simulink model "lab6"  (R2015a)
settings: Solver=ode45  StartTime=0.0  StopTime=500.0  MaxStep=0.2  RelTol=1e-3
values from neighbouring files (symbols this model uses):
  ddMax = 3    [lab6.m]
  deltaMax = 30    [lab6.m]
  fConst = 0    [lab6.m]
  K = 0.08    [lab6.m]
  Kaw = 2.604    [lab6.m]
  Kc = 1.04    [lab6.m]
  phiZad = 30    [lab6.m]
  Ti = 200    [lab6.m]
  Tr = 1    [lab6.m]
  Ts = 16.4    [lab6.m]
settings Model: Creator=vbox  LastModifiedBy=vbox
settings DataIOCC: InspectSignalLogs=on

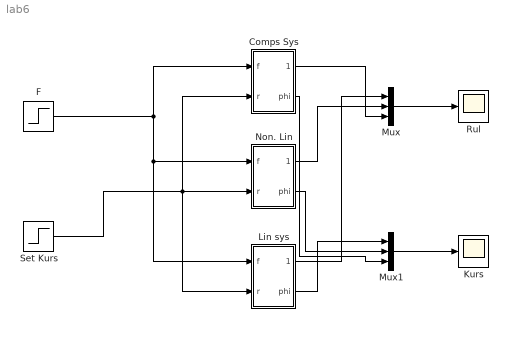
== system lab6 ==
  Comps Sys : Subsystem
  F : Step  After=fConst  SampleTime=0
  Kurs : Scope
      settings: SaveName=phi
  Lin sys : Subsystem
  Mux : Mux  Inputs=3
  Mux1 : Mux  Inputs=3
  Non. Lin : Subsystem
  Rul : Scope
      settings: TimeRange=100  YMin=0  YMax=400  SaveName=delta
  Set Kurs : Step  Time=0  After=phiZad  SampleTime=0
  wires:
  F/1 -> Non. Lin/1(f), Lin sys/1(f), Comps Sys/1(f)
  Set Kurs/1 -> Lin sys/2(r), Comps Sys/2(r), Non. Lin/2(r)
  Mux1/1 -> Kurs/1
  Mux/1 -> Rul/1
  Lin sys/1(delta) -> Mux/1
  Lin sys/2(phi) -> Mux1/1
  Non. Lin/1(delta) -> Mux/2
  Non. Lin/2(phi) -> Mux1/2
  Comps Sys/2(phi) -> Mux1/3
  Comps Sys/1(delta) -> Mux/3

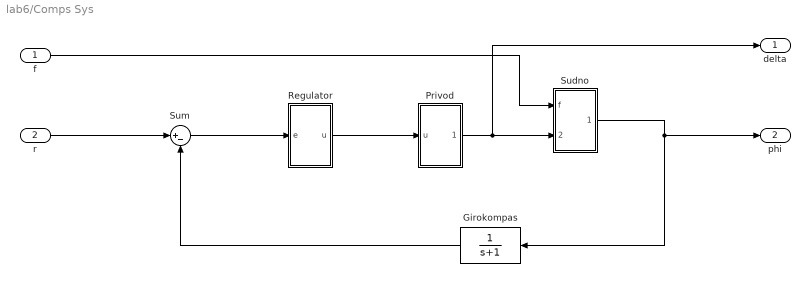
== system lab6/Comps Sys ==
  f : Inport
  r : Inport  Port=2
  Girokompas : TransferFcn  Denominator=[1 1]
  Privod : Subsystem
  Regulator : Subsystem
  Sudno : Subsystem
  Sum : Sum  Inputs=|+-
  delta : Outport
  phi : Outport  Port=2
  wires:
  Girokompas/1 -> Sum/2
  r/1 -> Sum/1
  Sudno/1(phi) -> phi/1, Girokompas/1
  Sum/1 -> Regulator/1(e)
  f/1 -> Sudno/1(f)
  Privod/1(delta) -> delta/1, Sudno/2(delta)
  Regulator/1(u) -> Privod/1(u)

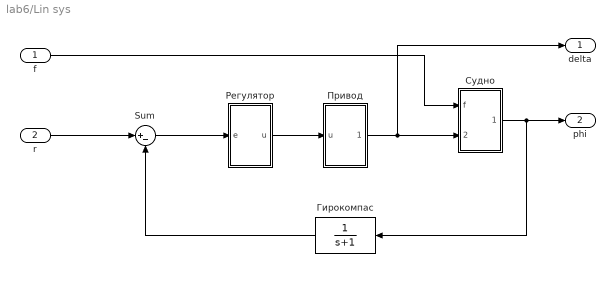
== system lab6/Lin sys ==
  f : Inport
  r : Inport  Port=2
  Sum : Sum  Inputs=|+-
  Гирокомпас : TransferFcn  Denominator=[1 1]
  Привод : Subsystem
  Регулятор : Subsystem
  Судно : Subsystem
  delta : Outport
  phi : Outport  Port=2
  wires:
  Гирокомпас/1 -> Sum/2
  r/1 -> Sum/1
  Судно/1(phi) -> phi/1, Гирокомпас/1
  Sum/1 -> Регулятор/1(e)
  f/1 -> Судно/1(f)
  Привод/1(delta) -> delta/1, Судно/2(delta)
  Регулятор/1(u) -> Привод/1(u)

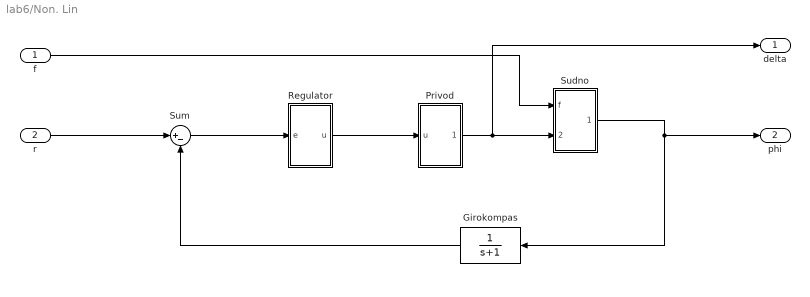
== system lab6/Non. Lin ==
  f : Inport
  r : Inport  Port=2
  Girokompas : TransferFcn  Denominator=[1 1]
  Privod : Subsystem
  Regulator : Subsystem
  Sudno : Subsystem
  Sum : Sum  Inputs=|+-
  delta : Outport
  phi : Outport  Port=2
  wires:
  Girokompas/1 -> Sum/2
  r/1 -> Sum/1
  Sudno/1(phi) -> phi/1, Girokompas/1
  Sum/1 -> Regulator/1(e)
  f/1 -> Sudno/1(f)
  Privod/1(delta) -> delta/1, Sudno/2(delta)
  Regulator/1(u) -> Privod/1(u)

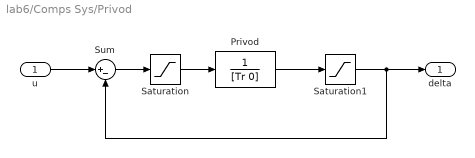
== system lab6/Comps Sys/Privod ==
  u : Inport
  Privod : TransferFcn  Denominator=[Tr 0]
  Saturation : Saturate  UpperLimit=Tr*ddMax  LowerLimit=-Tr*ddMax
      settings: LockScale=on
  Saturation1 : Saturate  UpperLimit=deltaMax  LowerLimit=-deltaMax
  Sum : Sum  Inputs=|+-
  delta : Outport
  wires:
  u/1 -> Sum/1
  Sum/1 -> Saturation/1
  Saturation/1 -> Privod/1
  Privod/1 -> Saturation1/1
  Saturation1/1 -> Sum/2, delta/1

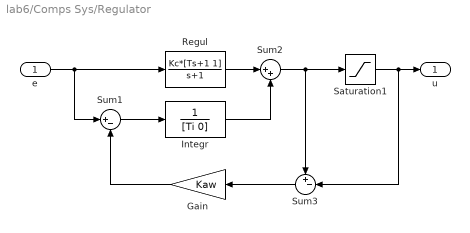
== system lab6/Comps Sys/Regulator ==
  e : Inport
  Gain : Gain  Gain=Kaw
  Integr : TransferFcn  Denominator=[Ti 0]
  Regul : TransferFcn  Numerator=Kc*[Ts+1 1]  Denominator=[1 1]
  Saturation1 : Saturate  UpperLimit=deltaMax  LowerLimit=-deltaMax
  Sum1 : Sum  Inputs=|+-
  Sum2 : Sum  Inputs=|++
  Sum3 : Sum  Inputs=+-|
  u : Outport
  wires:
  e/1 -> Sum1/1, Regul/1
  Regul/1 -> Sum2/1
  Integr/1 -> Sum2/2
  Sum1/1 -> Integr/1
  Sum2/1 -> Saturation1/1, Sum3/1
  Saturation1/1 -> Sum3/2, u/1
  Gain/1 -> Sum1/2
  Sum3/1 -> Gain/1

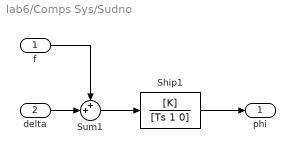
== system lab6/Comps Sys/Sudno ==
  f : Inport
  delta : Inport  Port=2
  Ship1 : TransferFcn  Numerator=[K]  Denominator=[Ts 1 0]
  Sum1 : Sum  Inputs=++|
  phi : Outport
  wires:
  Sum1/1 -> Ship1/1
  Ship1/1 -> phi/1
  f/1 -> Sum1/1
  delta/1 -> Sum1/2

== system lab6/Lin sys/Привод ==
  u : Inport
  привод : TransferFcn  Denominator=[Tr 1]
  delta : Outport
  wires:
  привод/1 -> delta/1
  u/1 -> привод/1

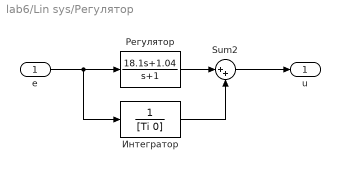
== system lab6/Lin sys/Регулятор ==
  e : Inport
  Sum2 : Sum  Inputs=|++
  Интегратор : TransferFcn  Denominator=[Ti 0]
  Регулятор : TransferFcn  Numerator=[18.1 1.04]  Denominator=[1 1]
  u : Outport
  wires:
  e/1 -> Интегратор/1, Регулятор/1
  Sum2/1 -> u/1
  Регулятор/1 -> Sum2/1
  Интегратор/1 -> Sum2/2

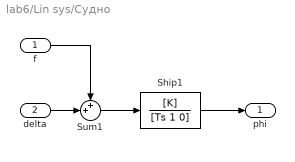
== system lab6/Lin sys/Судно ==
  f : Inport
  delta : Inport  Port=2
  Ship1 : TransferFcn  Numerator=[K]  Denominator=[Ts 1 0]
  Sum1 : Sum  Inputs=++|
  phi : Outport
  wires:
  Sum1/1 -> Ship1/1
  Ship1/1 -> phi/1
  f/1 -> Sum1/1
  delta/1 -> Sum1/2

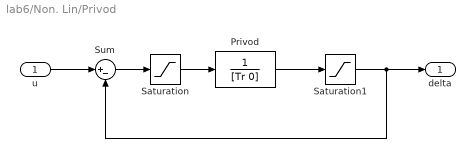
== system lab6/Non. Lin/Privod ==
  u : Inport
  Privod : TransferFcn  Denominator=[Tr 0]
  Saturation : Saturate  UpperLimit=Tr*ddMax  LowerLimit=-Tr*ddMax
      settings: LockScale=on
  Saturation1 : Saturate  UpperLimit=deltaMax  LowerLimit=-deltaMax
  Sum : Sum  Inputs=|+-
  delta : Outport
  wires:
  u/1 -> Sum/1
  Sum/1 -> Saturation/1
  Saturation/1 -> Privod/1
  Privod/1 -> Saturation1/1
  Saturation1/1 -> Sum/2, delta/1

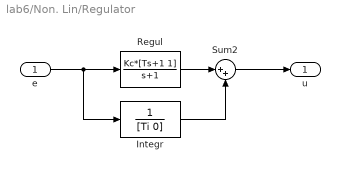
== system lab6/Non. Lin/Regulator ==
  e : Inport
  Integr : TransferFcn  Denominator=[Ti 0]
  Regul : TransferFcn  Numerator=Kc*[Ts+1 1]  Denominator=[1 1]
  Sum2 : Sum  Inputs=|++
  u : Outport
  wires:
  e/1 -> Integr/1, Regul/1
  Sum2/1 -> u/1
  Regul/1 -> Sum2/1
  Integr/1 -> Sum2/2

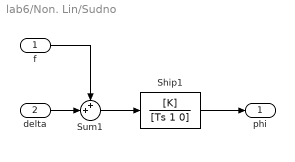
== system lab6/Non. Lin/Sudno ==
  f : Inport
  delta : Inport  Port=2
  Ship1 : TransferFcn  Numerator=[K]  Denominator=[Ts 1 0]
  Sum1 : Sum  Inputs=++|
  phi : Outport
  wires:
  Sum1/1 -> Ship1/1
  Ship1/1 -> phi/1
  f/1 -> Sum1/1
  delta/1 -> Sum1/2
